simulink model "attack2"  (R2021a)
settings: Solver=VariableStepAuto  StartTime=0.0  StopTime=20.0  RelTol=1e-3
settings Model: Creator=Suman  LastModifiedBy=Suman

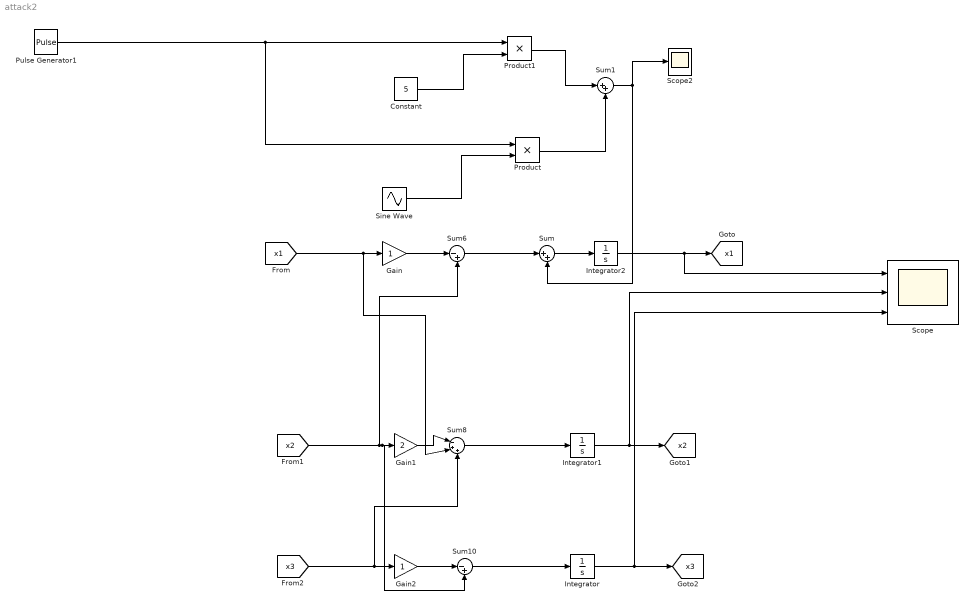
== system attack2 ==
  Constant : Constant  Value=5
  Gain : Gain
  Gain1 : Gain  Gain=2
  Gain2 : Gain
  Integrator : Integrator  InitialCondition=1
  Integrator1 : Integrator  InitialCondition=1
  Integrator2 : Integrator  InitialCondition=1
  Product : Product
  Product1 : Product
  Pulse Generator1 : DiscretePulseGenerator  PulseType=Time based  Period=20  PulseWidth=99.9999999  PhaseDelay=5
  Scope : Scope  NumInputPorts=3
  Scope2 : Scope
  Sine Wave : Sin  SampleTime=0.001
  Sum : Sum  Inputs=|++
  Sum1 : Sum  Inputs=|++
  Sum10 : Sum  Inputs=|-+
  Sum6 : Sum  Inputs=|-+
  Sum8 : Sum  Inputs=|-++
  tag scope: x1=global, x2=global, x3=global
  wires:
  Sum8/1 -> Integrator1/1
  Sum10/1 -> Integrator/1
  Gain2/1 -> Sum10/1
  Sum/1 -> Integrator2/1
  Gain1/1 -> Sum8/1
  [x3] -> Sum8/3, Gain2/1
  Gain/1 -> Sum6/1
  [x2] -> Sum10/2, Gain1/1, Sum6/2
  [x1] -> Sum8/2, Gain/1
  Sum6/1 -> Sum/1
  Sine Wave/1 -> Product/2
  Constant/1 -> Product1/2
  Product1/1 -> Sum1/1
  Product/1 -> Sum1/2
  Sum1/1 -> Sum/2, Scope2/1
  Pulse Generator1/1 -> Product/1, Product1/1
  Integrator/1 -> Scope/3, [x3]
  Integrator1/1 -> Scope/2, [x2]
  Integrator2/1 -> Scope/1, [x1]
